simulink model "simulink_lab_4"  (R2016b)
settings: Solver=ode4  StartTime=0.0  StopTime=40*T  FixedStep=T/1000  RelTol=1e-3
values from neighbouring files (symbols this model uses):
  C = 0.1*10^(-6)    (= 1e-07)    [circuitlab.m]    (also in matlabworckspace.mat)
  f = 2000    [circuitlab.m]    (also in matlabworckspace.mat)
  R1 = 4610    [circuitlab.m]    (also in matlabworckspace.mat)
  R2 = 46200    [circuitlab.m]    (also in matlabworckspace.mat)
settings Model: Creator=melabuser  LastModifiedBy=melabuser

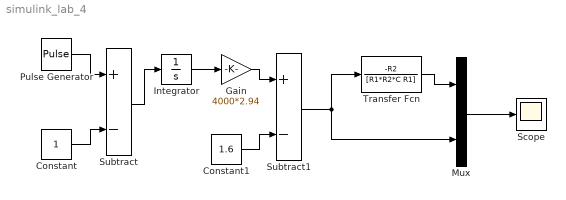
== system simulink_lab_4 ==
  Constant : Constant
  Constant1 : Constant  Value=1.6
  Gain : Gain  Gain=4000*2.94
  Integrator : Integrator
  Mux : Mux  Inputs=2
  Pulse Generator : DiscretePulseGenerator  PulseType=Time based  Amplitude=2  Period=1/f  PulseWidth=50
  Scope : Scope
  Subtract : Sum  Inputs=+-
  Subtract1 : Sum  Inputs=+-
  Transfer Fcn : TransferFcn  Numerator=-R2  Denominator=[R1*R2*C R1]
  wires:
  Constant/1 -> Subtract/2
  Transfer Fcn/1 -> Mux/1
  Mux/1 -> Scope/1
  Pulse Generator/1 -> Subtract/1
  Constant1/1 -> Subtract1/2
  Subtract/1 -> Integrator/1
  Integrator/1 -> Gain/1
  Gain/1 -> Subtract1/1
  Subtract1/1 -> Mux/2, Transfer Fcn/1
